simulink model "Project_3_Kinematic_Model"  (R2025a)
settings: Solver=VariableStepAuto  StartTime=0.0  StopTime=1400  RelTol=1e-3
undefined symbols (not defined in the file): carData, datMotor
libraries: SignalEditorBlockLib x1, slpidlib x1
settings Model: Creator=jr843  LastModifiedBy=jr843

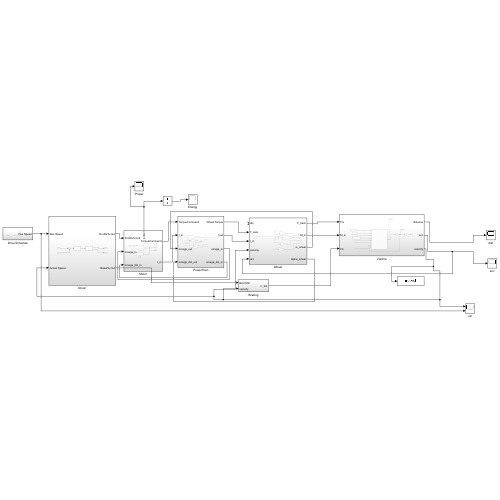
[thumbnail: Simulink's stored preview of the top-level diagram]
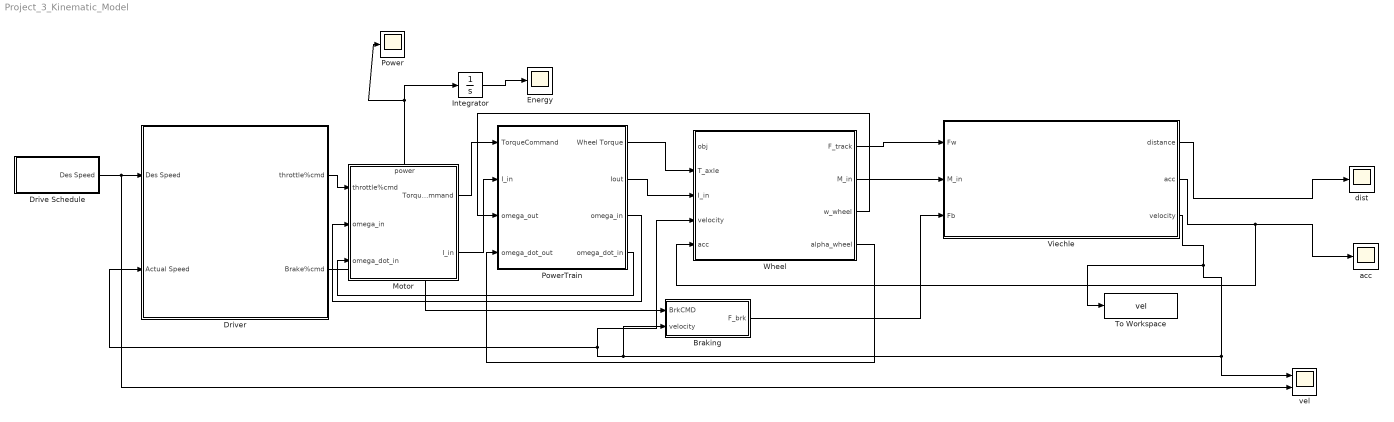
== system Project_3_Kinematic_Model ==
  Braking : Subsystem
  Drive Schedule : Subsystem
  Driver : Subsystem
  Energy : Scope
      settings: ActiveDisplayYMinimum=2.2641779954489432E+6  ActiveDisplayYMaximum=6.7863437137883417E+6  DataLoggingVariableName=ScopeData5
  Integrator : Integrator
  Motor : Subsystem
      settings: PortSchema="{\"entries\":[{\"content\":{\"sides\":[{\"content\":{\"connectorIds\":[\"In1\",\"In2\",\"In3\"]},\"type\":\"ConnectorPlacement.EquallySpacedRectSide\",\"uuid\":\"e82f964b-420f-4501-a544-50c992d60455\"},{\"content\":{\"connectorIds\":[\"Out1\",\"Out2\"],\"side\":\"RIGHT\"},\"type\":\"ConnectorPlacement.EquallySpacedRectSide\",\"uuid\":\"a73a6c5d-af26-4f75-8b6c-55b332079af1\"},{\"content\":{\"connectorIds\":[\"Out3\"],\"side\":\"TOP\"},\"type\":\"ConnectorPlacement.EquallySpacedRectSide\",\"uuid\":\"51f0513d-e736-4704-82f2-ea739249be70\"}]},\"type\":\"ConnectorPlacement.EquallySpacedConnector\",\"uuid\":\"5c632a6c-ac55-475e-b9a4-f1c9de387cb8\"}],\"packageUris\":[\"http://schema.mathworks.com/mf0/Connector/R2020b\"],\"version\":\"1.0\"}"
  Power : Scope
      settings: ActiveDisplayYMinimum=-56532.630229308081  ActiveDisplayYMaximum=508793.63918077317  DataLoggingVariableName=ScopeData4
  PowerTrain : Subsystem
  To Workspace : ToWorkspace  VariableName=vel  SaveFormat=Timeseries  SampleTime=-1
  Viechle : Subsystem
  Wheel : Subsystem
  acc : Scope
  dist : Scope
  vel : Scope  NumInputPorts=2
      settings: ActiveDisplayYMinimum=0.11510993568039574  ActiveDisplayYMaximum=21.142622084258356  DataLoggingVariableName=ScopeData2
  wires:
  Driver/2(Brake%cmd) -> Braking/1(BrkCMD)
  PowerTrain/1(Wheel Torque) -> Wheel/2(T_axle)
  PowerTrain/2(Iout) -> Wheel/3(I_in)
  Wheel/1(F_track) -> Viechle/1(Fw)
  Wheel/2(M_in) -> Viechle/2(M_in)
  Viechle/3(velocity) -> vel/1, Wheel/4(velocity), Driver/2(Actual Speed), Braking/2(velocity), To Workspace/1
  Braking/1(F_brk) -> Viechle/3(Fb)
  Drive Schedule/1(Des Speed) -> vel/2, Driver/1(Des Speed)
  Viechle/1(distance) -> dist/1
  Viechle/2(acc) -> Wheel/5(acc), acc/1
  Driver/1(throttle%cmd) -> Motor/1(throttle%cmd)
  Motor/1(TorqueCommand) -> PowerTrain/1(TorqueCommand)
  Motor/2(I_in) -> PowerTrain/2(I_in)
  Motor/3(power) -> Integrator/1, Power/1
  PowerTrain/3(omega_in) -> Motor/2(omega_in)
  PowerTrain/4(omega_dot_in) -> Motor/3(omega_dot_in)
  Wheel/3(w_wheel) -> PowerTrain/3(omega_out)
  Wheel/4(alpha_wheel) -> PowerTrain/4(omega_dot_out)
  Integrator/1 -> Energy/1

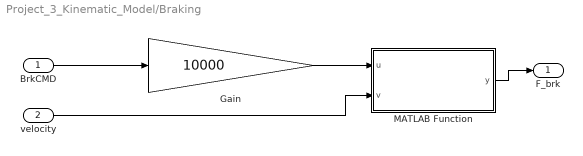
== system Project_3_Kinematic_Model/Braking ==
  BrkCMD : Inport
  velocity : Inport  Port=2
  Gain : Gain  Gain=10000
  MATLAB Function : MATLAB Function  TreatAsAtomicUnit=on
  F_brk : Outport
  wires:
  BrkCMD/1 -> Gain/1
  Gain/1 -> MATLAB Function/1(u)
  MATLAB Function/1(y) -> F_brk/1
  velocity/1 -> MATLAB Function/2(v)

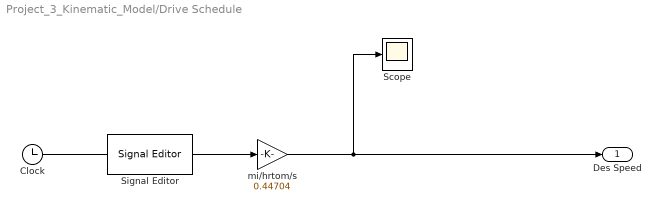
== system Project_3_Kinematic_Model/Drive Schedule ==
  Clock : Clock
  Scope : Scope
      settings: ActiveDisplayYMinimum=-3.1683959999999991  ActiveDisplayYMaximum=28.515564  DataLoggingVariableName=ScopeData3
  Signal Editor : SignalEditorBlockLib/Signal Editor  FileName=EPA_urban.mat  ActiveScenario=udds_columns  ActiveSignal=Speed  IsBus=off  OutputBusObjectStr=Bus: BusObject  SampleTime=1  ZeroCross=off  OutputAfterFinalValue=Setting to zero  Unit=mi/hr  PreserveSignalName=on  ApplySigPropsToAllScenarios=off  ApplySigPropsToAllSignals=on  SignalPropertySource=Dialog parameters
  mi/hrtom/s : Gain  Gain=0.44704
  Des Speed : Outport
  wires:
  mi/hrtom/s/1 -> Scope/1, Des Speed/1
  Signal Editor/1 -> mi/hrtom/s/1
  Clock/1 -> ?

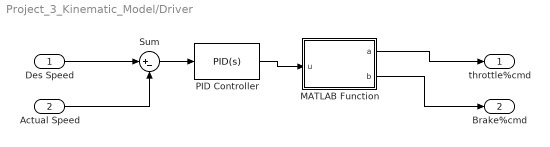
== system Project_3_Kinematic_Model/Driver ==
  Des Speed : Inport
  Actual Speed : Inport  Port=2
  MATLAB Function : MATLAB Function  TreatAsAtomicUnit=on
  PID Controller : slpidlib/PID Controller  Controller=PID  Form=Parallel  TimeDomain=Continuous-time  UseExternalTs=off  SampleTime=-1  IntegratorMethod=Forward Euler  FilterMethod=Forward Euler  ControllerParametersSource=internal  P=0.1  I=0  UseKiTs=off  D=0  UseExternalDerivativeSource=off  N=100  UseFilter=on  TunerSelectOption=Transfer Function Based (PID Tuner App)  InitialConditionSource=internal  InitialConditionForIntegrator=0  InitialConditionForFilter=0  DifferentiatorICPrevScaledInput=0  ExternalReset=none  TrackingMode=off  Kt=1  LimitOutput=on  SatLimitsSource=internal  UpperSaturationLimit=1  LowerSaturationLimit=-1  LinearizeAsGain=off  AntiWindupMode=none  Kb=1  LimitIntegrator=off  UpperIntegratorSaturationLimit=inf  LowerIntegratorSaturationLimit=-inf  POutMin=[]  POutMax=[]  IOutMin=[]  IOutMax=[]  DOutMin=[]  DOutMax=[]  NOutMin=[]  NOutMax=[]  SumOutMin=[]  SumOutMax=[]  SaturationOutMin=[]  SaturationOutMax=[]  PParamMin=[]  PParamMax=[]  IParamMin=[]  IParamMax=[]  DParamMin=[]  DParamMax=[]  NParamMin=[]  NParamMax=[]  KbParamMin=[]  KbParamMax=[]  KtParamMin=[]  KtParamMax=[]  KbOutMin=[]  KbOutMax=[]  KtOutMin=[]  KtOutMax=[]  IntegratorOutMin=[]  IntegratorOutMax=[]  FilterOutMin=[]  FilterOutMax=[]  SumI1OutMin=[]  SumI1OutMax=[]  SumI2OutMin=[]  SumI2OutMax=[]  SumI3OutMin=[]  SumI3OutMax=[]  SumI4OutMin=[]  SumI4OutMax=[]  SumDOutMin=[]  SumDOutMax=[]  DifferentiatorOutMin=[]  DifferentiatorOutMax=[]  FilterDiffOutCoefMin=[]  FilterDiffOutCoefMax=[]  ReciprocalOutMin=[]  ReciprocalOutMax=[]  SumDenOutMin=[]  SumDenOutMax=[]  SumNumOutMin=[]  SumNumOutMax=[]  DivideOutMin=[]  DivideOutMax=[]  UdiffTsProdOutMin=[]  UdiffTsProdOutMax=[]  NTsProdOutMin=[]  NTsProdOutMax=[]  UintegralTsProdOutMin=[]  UintegralTsProdOutMax=[]  UngainTsProdOutMin=[]  UngainTsProdOutMax=[]  ClampingZeroOutDataTypeStr=Inherit: Inherit via back propagation  ClampingZeroOutMin=[]  ClampingZeroOutMax=[]  FilterDenConstantOutDataTypeStr=Inherit: Inherit via back propagation  FilterDenConstantOutMin=[]  FilterDenConstantOutMax=[]  PCopyOutDataTypeStr=Inherit: Inherit via back propagation  PCopyOutMin=[]  PCopyOutMax=[]  NCopyOutDataTypeStr=Inherit: Inherit via back propagation  NCopyOutMin=[]  NCopyOutMax=[]  IntegratorContinuousStateAttributes=''  IntegratorStateMustResolveToSignalObject=off  IntegratorRTWStateStorageClass=Auto  FilterContinuousStateAttributes=''  FilterStateMustResolveToSignalObject=off  FilterRTWStateStorageClass=Auto  ParallelPVariant=InternalParameters  IdealPVariant=Disabled  IVariant=InternalParameters  DVariant=InternalParameters  IntegratorVariant=Continuous  SatVariant=Enabled  AWVariant=Passthrough  PCopyVariant=Disabled  TRVariant=Disabled  FdbkBlocksVariant=Forward  IdealPFdbkVariant=Disabled  SatFdbkVariant=Disabled  DerivativeFilterVariant=ContFilter  NVariant=InternalParameters  NCopyVariant=Disabled  FilterICVariant=InternalICsFilter  IntegratorICVariant=InternalICs  ExternalResetVariant=Disabled  TRSumVariant=Passthrough  SumFdbkVariant=Disabled  SumVariant=Sum_PID  TsampFilterVariant=InternalTs  TsampNgainVariant=Passthrough  TsampIntegralVariant=Disabled_SignalSpec  ExternalSaturationOutDataTypeStr=Inherit: Same as second input  DerivativeSourceVariant=ErrorSignal  PreIntVariant=InternalPreInt
  Sum : Sum  Inputs=|+-
  throttle%cmd : Outport
  Brake%cmd : Outport  Port=2
  wires:
  Actual Speed/1 -> Sum/2
  Des Speed/1 -> Sum/1
  Sum/1 -> PID Controller/1
  PID Controller/1 -> MATLAB Function/1(u)
  MATLAB Function/1(a) -> throttle%cmd/1
  MATLAB Function/2(b) -> Brake%cmd/1

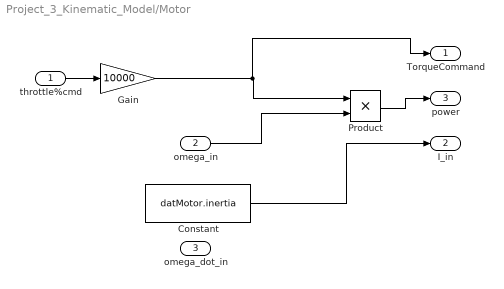
== system Project_3_Kinematic_Model/Motor ==
  throttle%cmd : Inport
  omega_in : Inport  Port=2
  omega_dot_in : Inport  Port=3
  Constant : Constant  Value=datMotor.inertia
  Gain : Gain  Gain=10000
  Product : Product
  TorqueCommand : Outport
  I_in : Outport  Port=2
  power : Outport  Port=3
  wires:
  omega_in/1 -> Product/2
  Product/1 -> power/1
  Constant/1 -> I_in/1
  Gain/1 -> TorqueCommand/1, Product/1
  throttle%cmd/1 -> Gain/1

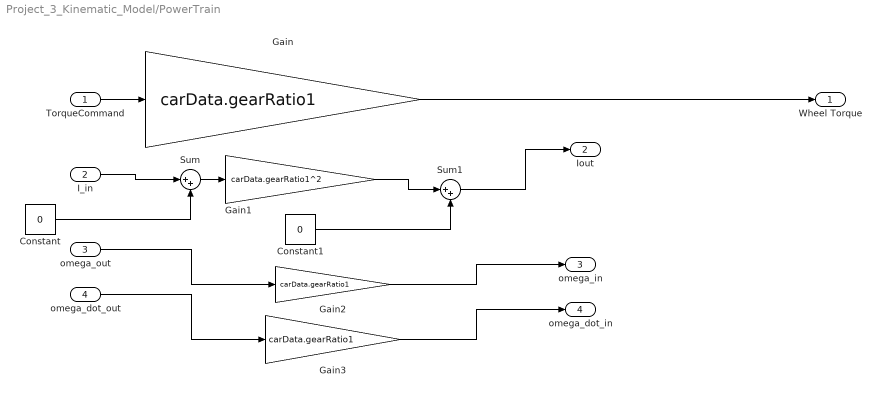
== system Project_3_Kinematic_Model/PowerTrain ==
  TorqueCommand : Inport
  I_in : Inport  Port=2
  omega_out : Inport  Port=3
  omega_dot_out : Inport  Port=4
  Constant : Constant  Value=0
  Constant1 : Constant  Value=0
  Gain : Gain  Gain=carData.gearRatio1
  Gain1 : Gain  Gain=carData.gearRatio1^2
  Gain2 : Gain  Gain=carData.gearRatio1
  Gain3 : Gain  Gain=carData.gearRatio1
  Sum : Sum  Inputs=|++
  Sum1 : Sum  Inputs=|++
  Wheel Torque : Outport
  Iout : Outport  Port=2
  omega_in : Outport  Port=3
  omega_dot_in : Outport  Port=4
  wires:
  TorqueCommand/1 -> Gain/1
  I_in/1 -> Sum/1
  Constant/1 -> Sum/2
  Sum/1 -> Gain1/1
  Gain1/1 -> Sum1/1
  Constant1/1 -> Sum1/2
  Sum1/1 -> Iout/1
  omega_dot_out/1 -> Gain3/1
  Gain3/1 -> omega_dot_in/1
  Gain2/1 -> omega_in/1
  omega_out/1 -> Gain2/1
  Gain/1 -> Wheel Torque/1

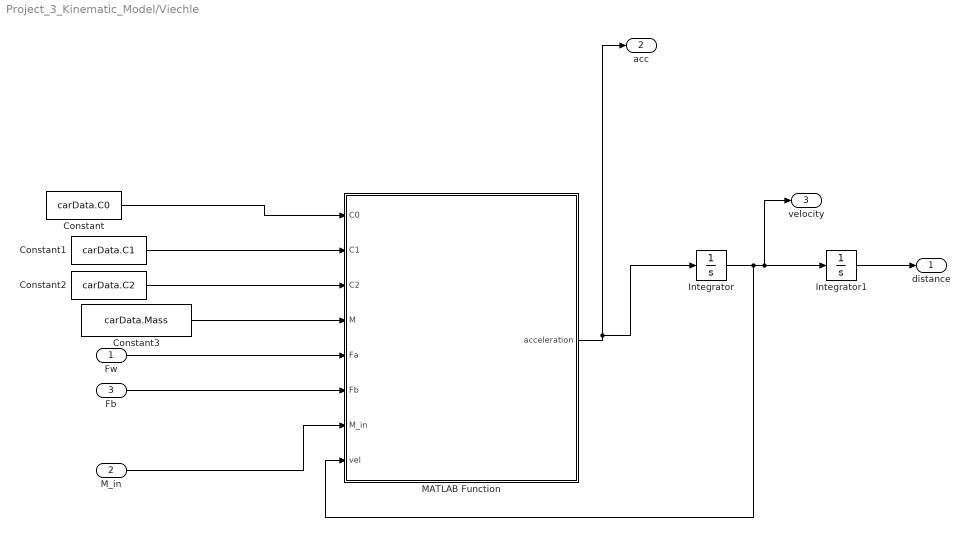
== system Project_3_Kinematic_Model/Viechle ==
  Fw : Inport
  M_in : Inport  Port=2
  Fb : Inport  Port=3
  Constant : Constant  Value=carData.C0
  Constant1 : Constant  Value=carData.C1
  Constant2 : Constant  Value=carData.C2
  Constant3 : Constant  Value=carData.Mass
  Integrator : Integrator
  Integrator1 : Integrator
  MATLAB Function : MATLAB Function  TreatAsAtomicUnit=on
  distance : Outport
  acc : Outport  Port=2
  velocity : Outport  Port=3
  wires:
  Constant/1 -> MATLAB Function/1(C0)
  Constant1/1 -> MATLAB Function/2(C1)
  Constant2/1 -> MATLAB Function/3(C2)
  Constant3/1 -> MATLAB Function/4(M)
  Fw/1 -> MATLAB Function/5(Fa)
  Fb/1 -> MATLAB Function/6(Fb)
  M_in/1 -> MATLAB Function/7(M_in)
  MATLAB Function/1(acceleration) -> Integrator/1, acc/1
  Integrator/1 -> MATLAB Function/8(vel), velocity/1, Integrator1/1
  Integrator1/1 -> distance/1

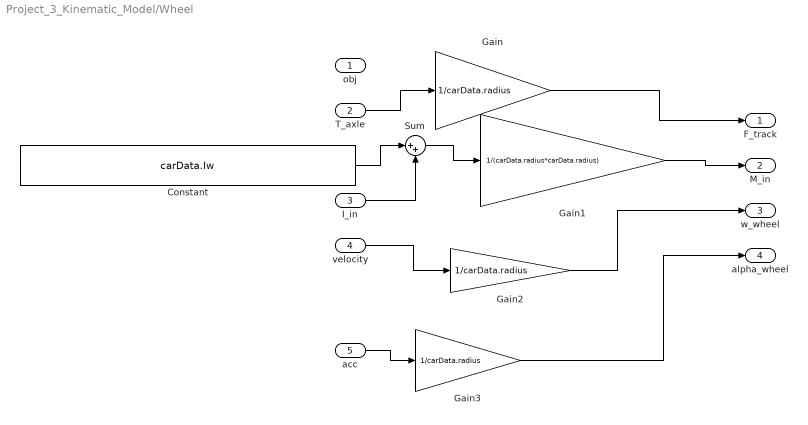
== system Project_3_Kinematic_Model/Wheel ==
  obj : Inport
  T_axle : Inport  Port=2
  I_in : Inport  Port=3
  velocity : Inport  Port=4
  acc : Inport  Port=5
  Constant : Constant  Value=carData.Iw
  Gain : Gain  Gain=1/carData.radius
  Gain1 : Gain  Gain=1/(carData.radius*carData.radius)
  Gain2 : Gain  Gain=1/carData.radius
  Gain3 : Gain  Gain=1/carData.radius
  Sum : Sum  Inputs=|++
  F_track : Outport
  M_in : Outport  Port=2
  w_wheel : Outport  Port=3
  alpha_wheel : Outport  Port=4
  wires:
  T_axle/1 -> Gain/1
  Gain/1 -> F_track/1
  Constant/1 -> Sum/1
  I_in/1 -> Sum/2
  Sum/1 -> Gain1/1
  Gain1/1 -> M_in/1
  velocity/1 -> Gain2/1
  Gain2/1 -> w_wheel/1
  acc/1 -> Gain3/1
  Gain3/1 -> alpha_wheel/1

== matlab function Project_3_Kinematic_Model/Driver/MATLAB Function ==
  data: u input; a output; b output
function [a,b] = fcn(u)

if u>0
    acc=u;
    brk=0;
elseif u<0
    acc=0;
    brk=-u;
else
    acc=0;
    brk=0;
end
a=acc;
b=brk;

== matlab function Project_3_Kinematic_Model/Braking/MATLAB Function ==
  data: u input; y output; v input
function y = fcn(u, v)

%y=usign(v)
y=u*v/(abs(v)+0.001);
y = u;

== matlab function Project_3_Kinematic_Model/Viechle/MATLAB Function ==
  data: C0 input; acceleration output; C1 input; C2 input; M input; Fa input; Fb input; M_in input; vel input
function acceleration = fcn(C0, C1, C2, M, Fa, Fb, M_in, vel)

acceleration = (((Fa-Fb))-(C0+C1*vel+C2*(vel)^2))/(M+M_in);
